simulink model "EV_Modeling_old"  (R2024b)
settings: Solver=FixedStepAuto  StartTime=0.0  StopTime=10382  FixedStep=0.1  RelTol=1e-3
values from neighbouring files (symbols this model uses):
  battery_SOC_SOC = battery_SOC(:,1)    [EV_Truck.m]    (also in simulink.m)
  battery_SOC_voltage = battery_SOC(:,2)    [EV_Truck.m]    (also in simulink.m)
  drag_coefficient_FV1 = table2array(drag_coefficient(:,3))    [simulink.m]
  drag_coefficient_FV2 = table2array(drag_coefficient(:,4))    [simulink.m]
  drag_coefficient_input = table2array(drag_coefficient(:,1))    [simulink.m]
  drag_coefficient_LV = table2array(drag_coefficient(:,2))    [simulink.m]
  electric_consumption_ressistancce = electric_consumption(:,2)    [EV_Truck.m]    (also in simulink.m)
  electric_consumption_voltage = electric_consumption(:,1)    [EV_Truck.m]    (also in simulink.m)
  motor_efficiency_efficiency = table2array(motor_efficiency(2:height(motor_efficiency),2:width(motor_efficiency)))    [EV_Truck.m]    (also in simulink.m)
  motor_efficiency_RPM = table2array(motor_efficiency(2:height(motor_efficiency),1))    [EV_Truck.m]    (also in simulink.m)
  motor_efficiency_torque = transpose(motor_efficiency_torque)    [EV_Truck.m]    (also in simulink.m)
  motor_RPM_torque = table2array(motor_torque(1:14,1))    [EV_Truck.m]    (also in simulink.m)
  motor_torque_RPM = table2array(motor_torque(1:14,2))    [EV_Truck.m]    (also in simulink.m)
undefined symbols (not defined in the file or in its folder): battery_builder_rtmsupport, battery_sli_rtmsupport, C1_mat, C2_mat, c_sqrt, DiscIntNeverNeededParam, dV0_mat, gcbh, n, Wc, Wm, x0
libraries: simulink x87, packLibrary_lib x30, nesl_utility x6, fl_lib x6, simulink_extras x3, mpcadaslib x2, slpidlib x1
(part 11 of 12)

== system EV_Modeling_old/FV2/SOC Estimator (Kalman Filter)1/Kalman Filter/UKF/Prediction/Measurement function ==
  Current : Inport
  Temperature : Inport  Port=2
  X : Inport  Port=3  Partition=on  PartitionDimension=2  PartitionWidth=1  PartitionOffset=0
  Constant : Constant  Value=Wm  OutDataTypeStr=Inherit: Inherit via back propagation
  Data Type Conversion Inherited : simulink/Signal Attributes/Data Type Conversion Inherited  ConvertRealWorld=Real World Value  DoSatur=off
  For Each : ForEach  DisableCoverage=on  ShowIterationIndex=on
  Measurement function : Subsystem
  Product : Product
  Selector : Selector  IndexMode=Zero-based  InputPortWidth=2*n+1  IndexOptions=Index vector (port)  Indices=[1 3]  OutputSizes=1
  y : Outport  ConcatenationDimension=2
  Wm_i*y_i : Outport  Port=2  SampleTime=Ts  ConcatenationDimension=2
  wires:
  Product/1 -> Wm_i*y_i/1
  Selector/1 -> Product/1
  For Each/1 -> Selector/2
  Measurement function/1(y) -> Product/2, y/1
  Temperature/1 -> Measurement function/2(Temperature)
  Current/1 -> Data Type Conversion Inherited/1, Measurement function/1(Current)
  X/1 -> Measurement function/3(x)
  Data Type Conversion Inherited/1 -> Selector/1
  Constant/1 -> Data Type Conversion Inherited/2

== system EV_Modeling_old/FV2/SOC Estimator (Kalman Filter)1/Kalman Filter/UKF/Prediction/State function ==
  Current : Inport
  Temperature : Inport  Port=2
  X : Inport  Port=3  Partition=on  PartitionDimension=2  PartitionWidth=1  PartitionOffset=0
  Constant : Constant  Value=Wm  OutDataTypeStr=Inherit: Inherit via back propagation
  Data Type Conversion Inherited : simulink/Signal Attributes/Data Type Conversion Inherited  ConvertRealWorld=Real World Value  DoSatur=off
  For Each : ForEach  DisableCoverage=on  ShowIterationIndex=on
  Product : Product
  Selector : Selector  IndexMode=Zero-based  InputPortWidth=2*n+1  IndexOptions=Index vector (port)  Indices=[1 3]  OutputSizes=1
  State function : Subsystem
  xk1 : Outport  ConcatenationDimension=2
  Wm_i*xk1_i : Outport  Port=2  SampleTime=Ts  ConcatenationDimension=2
  wires:
  X/1 -> State function/3(x)
  Current/1 -> Data Type Conversion Inherited/1, State function/1(Current)
  Temperature/1 -> State function/2(Temperature)
  State function/1(xk1) -> Product/2, xk1/1
  For Each/1 -> Selector/2
  Selector/1 -> Product/1
  Product/1 -> Wm_i*xk1_i/1
  Data Type Conversion Inherited/1 -> Selector/1
  Constant/1 -> Data Type Conversion Inherited/2

== system EV_Modeling_old/FV2/SOC Estimator (Kalman Filter)1/Kalman Filter/UKF 2RC/Prediction/Measurement function ==
  Current : Inport
  Temperature : Inport  Port=2
  X : Inport  Port=3  Partition=on  PartitionDimension=2  PartitionWidth=1  PartitionOffset=0
  Constant : Constant  Value=Wm  OutDataTypeStr=Inherit: Inherit via back propagation
  Data Type Conversion Inherited : simulink/Signal Attributes/Data Type Conversion Inherited  ConvertRealWorld=Real World Value  DoSatur=off
  For Each : ForEach  DisableCoverage=on  ShowIterationIndex=on
  Measurement function : Subsystem
  Product : Product
  Selector : Selector  IndexMode=Zero-based  InputPortWidth=2*n+1  IndexOptions=Index vector (port)  Indices=[1 3]  OutputSizes=1
  y : Outport  ConcatenationDimension=2
  Wm_i*y_i : Outport  Port=2  SampleTime=Ts  ConcatenationDimension=2
  wires:
  Product/1 -> Wm_i*y_i/1
  Selector/1 -> Product/1
  For Each/1 -> Selector/2
  Measurement function/1(y) -> Product/2, y/1
  Temperature/1 -> Measurement function/2(Temperature)
  Current/1 -> Data Type Conversion Inherited/1, Measurement function/1(Current)
  X/1 -> Measurement function/3(x)
  Data Type Conversion Inherited/1 -> Selector/1
  Constant/1 -> Data Type Conversion Inherited/2

== system EV_Modeling_old/FV2/SOC Estimator (Kalman Filter)1/Kalman Filter/UKF 2RC/Prediction/State function ==
  Current : Inport
  Temperature : Inport  Port=2
  X : Inport  Port=3  Partition=on  PartitionDimension=2  PartitionWidth=1  PartitionOffset=0
  Constant : Constant  Value=Wm  OutDataTypeStr=Inherit: Inherit via back propagation
  Data Type Conversion Inherited : simulink/Signal Attributes/Data Type Conversion Inherited  ConvertRealWorld=Real World Value  DoSatur=off
  For Each : ForEach  DisableCoverage=on  ShowIterationIndex=on
  Product : Product
  Selector : Selector  IndexMode=Zero-based  InputPortWidth=2*n+1  IndexOptions=Index vector (port)  Indices=[1 3]  OutputSizes=1
  State function : Subsystem
  xk1 : Outport  ConcatenationDimension=2
  Wm_i*xk1_i : Outport  Port=2  SampleTime=Ts  ConcatenationDimension=2
  wires:
  X/1 -> State function/3(x)
  Current/1 -> Data Type Conversion Inherited/1, State function/1(Current)
  Temperature/1 -> State function/2(Temperature)
  State function/1(xk1) -> Product/2, xk1/1
  For Each/1 -> Selector/2
  Selector/1 -> Product/1
  Product/1 -> Wm_i*xk1_i/1
  Data Type Conversion Inherited/1 -> Selector/1
  Constant/1 -> Data Type Conversion Inherited/2

== system EV_Modeling_old/LV/SOC Estimator (Kalman Filter)/Kalman Filter/UKBF/Prediction-correction/Measurement function ==
  Current : Inport
  Temperature : Inport  Port=2
  X : Inport  Port=3  Partition=on  PartitionDimension=2  PartitionWidth=1  PartitionOffset=0
  Constant : Constant  Value=Wm
  For Each : ForEach  DisableCoverage=on  ShowIterationIndex=on
  Measurement function : Subsystem
  Product : Product
  Selector : Selector  IndexMode=Zero-based  InputPortWidth=2*n+1  IndexOptions=Index vector (port)  Indices=[1 3]  OutputSizes=1
  h(X) : Outport  ConcatenationDimension=2
  h(X)*Wm : Outport  Port=2  ConcatenationDimension=2
  wires:
  Temperature/1 -> Measurement function/2(Temperature)
  Current/1 -> Measurement function/1(Current)
  X/1 -> Measurement function/3(x)
  For Each/1 -> Selector/2
  Constant/1 -> Selector/1
  Selector/1 -> Product/1
  Measurement function/1(y) -> Product/2, h(X)/1
  Product/1 -> h(X)*Wm/1

== system EV_Modeling_old/LV/SOC Estimator (Kalman Filter)/Kalman Filter/UKBF/Prediction-correction/State function ==
  Current : Inport
  Temperature : Inport  Port=2
  X : Inport  Port=3  Partition=on  PartitionDimension=2  PartitionWidth=1  PartitionOffset=0
  Constant : Constant  Value=double(Wm)
  For Each : ForEach  DisableCoverage=on  ShowIterationIndex=on
  Product : Product
  Product1 : Product
  Selector : Selector  IndexMode=Zero-based  InputPortWidth=2*n+1  IndexOptions=Index vector (port)  Indices=[1 3]  OutputSizes=1
  State function : Subsystem
  f(X) : Outport  ConcatenationDimension=2
  f(X)*Wm : Outport  Port=2  ConcatenationDimension=2
  X*Wm : Outport  Port=3  ConcatenationDimension=2
  wires:
  Current/1 -> State function/1(Current)
  Temperature/1 -> State function/2(Temperature)
  Constant/1 -> Selector/1
  Product/1 -> f(X)*Wm/1
  State function/1(f(x)) -> Product/2, f(X)/1
  Selector/1 -> Product1/1, Product/1
  For Each/1 -> Selector/2
  X/1 -> Product1/2, State function/3(x)
  Product1/1 -> X*Wm/1

== system EV_Modeling_old/LV/SOC Estimator (Kalman Filter)/Kalman Filter/UKBF/Prediction-correction/Update A ==
  X : Inport
  Constant : Constant  Value=ones(1,2*n+1)  VectorParams1D=off
  Gain : Gain  Gain=1/c_sqrt
  Matrix Multiply : Product  Multiplication=Matrix(*)
  Selector : Selector  NumberOfDimensions=2  InputPortWidth=3  IndexOptions=Index vector (dialog),Index vector (dialog)  Indices=[1:n],1  OutputSizes=1,1
  Selector1 : Selector  NumberOfDimensions=2  InputPortWidth=3  IndexOptions=Index vector (dialog),Index vector (dialog)  Indices=1:n,2:n+1  OutputSizes=1,1
  Sum : Sum  Inputs=|+-
  A(t) : Outport
  xhat : Outport  Port=2
  wires:
  X/1 -> Selector/1, Sum/1
  Selector/1 -> xhat/1, Matrix Multiply/1
  Constant/1 -> Matrix Multiply/2
  Matrix Multiply/1 -> Sum/2
  Sum/1 -> Gain/1
  Gain/1 -> Selector1/1
  Selector1/1 -> A(t)/1

== system EV_Modeling_old/LV/SOC Estimator (Kalman Filter)/Kalman Filter/UKBF/Prediction-correction/Xdot ==
  Voltage : Inport
  h(X) : Inport  Port=2
  mh : Inport  Port=3
  f(X) : Inport  Port=4
  mf : Inport  Port=5
  mx : Inport  Port=6
  X : Inport  Port=7
  A : Inport  Port=8
  Constant : Constant  Value=ones(1,2*n+1)  VectorParams1D=off
  Constant2 : Constant  Value=double(R)
  Constant3 : Constant  Value=eye(size(R,1))
  Divide : Product  Inputs=*/  Multiplication=Matrix(*)
  Gain3 : Gain  Gain=[Wc;Wc]
  Gain4 : Gain  Gain=[Wc;Wc]
  Matrix Multiply{,1..6,9} (8 alike) : Product  Multiplication=Matrix(*)
  Sigma points derivatives : Subsystem
  Sum : Sum  Inputs=|+-
  Sum1 : Sum  Inputs=|+-
  Sum2 : Sum  Inputs=|+-
  Sum4 : Sum  Inputs=-+|
  Sum5 : Sum
  Transpose : Math  Operator=transpose
  Transpose1 : Math  Operator=transpose
  Transpose2 : Math  Operator=transpose
  Update Fi : Subsystem
  Xdot : Outport
  wires:
  Constant/1 -> Matrix Multiply/2, Matrix Multiply1/2, Matrix Multiply2/2
  X/1 -> Sum/1
  f(X)/1 -> Sum1/1
  mf/1 -> Matrix Multiply1/1, Sum5/1
  h(X)/1 -> Sum2/1
  mh/1 -> Sum4/1, Matrix Multiply2/1
  Matrix Multiply/1 -> Sum/2
  Matrix Multiply1/1 -> Sum1/2
  Sum1/1 -> Gain4/1, Transpose/1
  Transpose/1 -> Matrix Multiply3/2
  Gain3/1 -> Matrix Multiply5/1, Matrix Multiply3/1
  Matrix Multiply2/1 -> Sum2/2
  Gain4/1 -> Matrix Multiply4/1
  Sum/1 -> Transpose1/1, Gain3/1
  Transpose1/1 -> Matrix Multiply4/2
  Sum2/1 -> Transpose2/1
  Transpose2/1 -> Matrix Multiply5/2
  Matrix Multiply5/1 -> Matrix Multiply6/1  "XWh"
  Constant2/1 -> Divide/2
  Constant3/1 -> Divide/1
  Divide/1 -> Matrix Multiply6/2
  Matrix Multiply6/1 -> Update Fi/4(K), Matrix Multiply9/1  "K"
  Voltage/1 -> Sum4/2
  Sum4/1 -> Matrix Multiply9/2
  Matrix Multiply9/1 -> Sum5/2
  Sum5/1 -> Sigma points derivatives/3(x1)
  A/1 -> Sigma points derivatives/1(A), Update Fi/1(A)
  Matrix Multiply3/1 -> Update Fi/2(XWf)  "XWf"
  Matrix Multiply4/1 -> Update Fi/3(fWX)  "fWX"
  Sigma points derivatives/1(Xdot) -> Xdot/1
  Update Fi/1(Fi) -> Sigma points derivatives/2(Fi)
  mx/1 -> Matrix Multiply/1

== system EV_Modeling_old/LV/SOC Estimator (Kalman Filter)/Kalman Filter/UKBF 2RC/Prediction-correction/Measurement function ==
  Current : Inport
  Temperature : Inport  Port=2
  X : Inport  Port=3  Partition=on  PartitionDimension=2  PartitionWidth=1  PartitionOffset=0
  Constant : Constant  Value=Wm
  For Each : ForEach  DisableCoverage=on  ShowIterationIndex=on
  Measurement function : Subsystem
  Product : Product
  Selector : Selector  IndexMode=Zero-based  InputPortWidth=2*n+1  IndexOptions=Index vector (port)  Indices=[1 3]  OutputSizes=1
  h(X) : Outport  ConcatenationDimension=2
  h(X)*Wm : Outport  Port=2  ConcatenationDimension=2
  wires:
  Temperature/1 -> Measurement function/2(Temperature)
  Current/1 -> Measurement function/1(Current)
  X/1 -> Measurement function/3(x)
  For Each/1 -> Selector/2
  Constant/1 -> Selector/1
  Selector/1 -> Product/1
  Measurement function/1(y) -> Product/2, h(X)/1
  Product/1 -> h(X)*Wm/1

== system EV_Modeling_old/LV/SOC Estimator (Kalman Filter)/Kalman Filter/UKBF 2RC/Prediction-correction/State function ==
  Current : Inport
  Temperature : Inport  Port=2
  X : Inport  Port=3  Partition=on  PartitionDimension=2  PartitionWidth=1  PartitionOffset=0
  Constant : Constant  Value=double(Wm)
  For Each : ForEach  DisableCoverage=on  ShowIterationIndex=on
  Product : Product
  Product1 : Product
  Selector : Selector  IndexMode=Zero-based  InputPortWidth=2*n+1  IndexOptions=Index vector (port)  Indices=[1 3]  OutputSizes=1
  State function : Subsystem
  f(X) : Outport  ConcatenationDimension=2
  f(X)*Wm : Outport  Port=2  ConcatenationDimension=2
  X*Wm : Outport  Port=3  ConcatenationDimension=2
  wires:
  Current/1 -> State function/1(Current)
  Temperature/1 -> State function/2(Temperature)
  Constant/1 -> Selector/1
  Product/1 -> f(X)*Wm/1
  State function/1(f(x)) -> Product/2, f(X)/1
  Selector/1 -> Product1/1, Product/1
  For Each/1 -> Selector/2
  X/1 -> Product1/2, State function/3(x)
  Product1/1 -> X*Wm/1

== system EV_Modeling_old/LV/SOC Estimator (Kalman Filter)/Kalman Filter/UKBF 2RC/Prediction-correction/Update A ==
  X : Inport
  Constant : Constant  Value=ones(1,2*n+1)  VectorParams1D=off
  Gain : Gain  Gain=1/c_sqrt
  Matrix Multiply : Product  Multiplication=Matrix(*)
  Selector : Selector  NumberOfDimensions=2  InputPortWidth=3  IndexOptions=Index vector (dialog),Index vector (dialog)  Indices=[1:n],1  OutputSizes=1,1
  Selector1 : Selector  NumberOfDimensions=2  InputPortWidth=3  IndexOptions=Index vector (dialog),Index vector (dialog)  Indices=1:n,2:n+1  OutputSizes=1,1
  Sum : Sum  Inputs=|+-
  A(t) : Outport
  xhat : Outport  Port=2
  wires:
  X/1 -> Selector/1, Sum/1
  Selector/1 -> xhat/1, Matrix Multiply/1
  Constant/1 -> Matrix Multiply/2
  Matrix Multiply/1 -> Sum/2
  Sum/1 -> Gain/1
  Gain/1 -> Selector1/1
  Selector1/1 -> A(t)/1

== system EV_Modeling_old/LV/SOC Estimator (Kalman Filter)/Kalman Filter/UKBF 2RC/Prediction-correction/Xdot ==
  Voltage : Inport
  h(X) : Inport  Port=2
  mh : Inport  Port=3
  f(X) : Inport  Port=4
  mf : Inport  Port=5
  mx : Inport  Port=6
  X : Inport  Port=7
  A : Inport  Port=8
  Constant : Constant  Value=ones(1,2*n+1)  VectorParams1D=off
  Constant2 : Constant  Value=double(R)
  Constant3 : Constant  Value=eye(size(R,1))
  Divide : Product  Inputs=*/  Multiplication=Matrix(*)
  Gain3 : Gain  Gain=[Wc;Wc;Wc]
  Gain4 : Gain  Gain=[Wc;Wc;Wc]
  Matrix Multiply{,1..6,9} (8 alike) : Product  Multiplication=Matrix(*)
  Sigma points derivatives : Subsystem
  Sum : Sum  Inputs=|+-
  Sum1 : Sum  Inputs=|+-
  Sum2 : Sum  Inputs=|+-
  Sum4 : Sum  Inputs=-+|
  Sum5 : Sum
  Transpose : Math  Operator=transpose
  Transpose1 : Math  Operator=transpose
  Transpose2 : Math  Operator=transpose
  Update Fi : Subsystem
  Xdot : Outport
  wires:
  Constant/1 -> Matrix Multiply/2, Matrix Multiply1/2, Matrix Multiply2/2
  X/1 -> Sum/1
  f(X)/1 -> Sum1/1
  mf/1 -> Matrix Multiply1/1, Sum5/1
  h(X)/1 -> Sum2/1
  mh/1 -> Sum4/1, Matrix Multiply2/1
  Matrix Multiply/1 -> Sum/2
  Matrix Multiply1/1 -> Sum1/2
  Sum1/1 -> Gain4/1, Transpose/1
  Transpose/1 -> Matrix Multiply3/2
  Gain3/1 -> Matrix Multiply5/1, Matrix Multiply3/1
  Matrix Multiply2/1 -> Sum2/2
  Gain4/1 -> Matrix Multiply4/1
  Sum/1 -> Transpose1/1, Gain3/1
  Transpose1/1 -> Matrix Multiply4/2
  Sum2/1 -> Transpose2/1
  Transpose2/1 -> Matrix Multiply5/2
  Matrix Multiply5/1 -> Matrix Multiply6/1  "XWh"
  Constant2/1 -> Divide/2
  Constant3/1 -> Divide/1
  Divide/1 -> Matrix Multiply6/2
  Matrix Multiply6/1 -> Update Fi/4(K), Matrix Multiply9/1  "K"
  Voltage/1 -> Sum4/2
  Sum4/1 -> Matrix Multiply9/2
  Matrix Multiply9/1 -> Sum5/2
  Sum5/1 -> Sigma points derivatives/3(x1)
  A/1 -> Sigma points derivatives/1(A), Update Fi/1(A)
  Matrix Multiply3/1 -> Update Fi/2(XWf)  "XWf"
  Matrix Multiply4/1 -> Update Fi/3(fWX)  "fWX"
  Sigma points derivatives/1(Xdot) -> Xdot/1
  Update Fi/1(Fi) -> Sigma points derivatives/2(Fi)
  mx/1 -> Matrix Multiply/1

== system EV_Modeling_old/LV/SOC Estimator (Kalman Filter)/Kalman Filter/UKF/Prediction/Measurement function ==
  Current : Inport
  Temperature : Inport  Port=2
  X : Inport  Port=3  Partition=on  PartitionDimension=2  PartitionWidth=1  PartitionOffset=0
  Constant : Constant  Value=Wm  OutDataTypeStr=Inherit: Inherit via back propagation
  Data Type Conversion Inherited : simulink/Signal Attributes/Data Type Conversion Inherited  ConvertRealWorld=Real World Value  DoSatur=off
  For Each : ForEach  DisableCoverage=on  ShowIterationIndex=on
  Measurement function : Subsystem
  Product : Product
  Selector : Selector  IndexMode=Zero-based  InputPortWidth=2*n+1  IndexOptions=Index vector (port)  Indices=[1 3]  OutputSizes=1
  y : Outport  ConcatenationDimension=2
  Wm_i*y_i : Outport  Port=2  SampleTime=Ts  ConcatenationDimension=2
  wires:
  Product/1 -> Wm_i*y_i/1
  Selector/1 -> Product/1
  For Each/1 -> Selector/2
  Measurement function/1(y) -> Product/2, y/1
  Temperature/1 -> Measurement function/2(Temperature)
  Current/1 -> Data Type Conversion Inherited/1, Measurement function/1(Current)
  X/1 -> Measurement function/3(x)
  Data Type Conversion Inherited/1 -> Selector/1
  Constant/1 -> Data Type Conversion Inherited/2

== system EV_Modeling_old/LV/SOC Estimator (Kalman Filter)/Kalman Filter/UKF/Prediction/State function ==
  Current : Inport
  Temperature : Inport  Port=2
  X : Inport  Port=3  Partition=on  PartitionDimension=2  PartitionWidth=1  PartitionOffset=0
  Constant : Constant  Value=Wm  OutDataTypeStr=Inherit: Inherit via back propagation
  Data Type Conversion Inherited : simulink/Signal Attributes/Data Type Conversion Inherited  ConvertRealWorld=Real World Value  DoSatur=off
  For Each : ForEach  DisableCoverage=on  ShowIterationIndex=on
  Product : Product
  Selector : Selector  IndexMode=Zero-based  InputPortWidth=2*n+1  IndexOptions=Index vector (port)  Indices=[1 3]  OutputSizes=1
  State function : Subsystem
  xk1 : Outport  ConcatenationDimension=2
  Wm_i*xk1_i : Outport  Port=2  SampleTime=Ts  ConcatenationDimension=2
  wires:
  X/1 -> State function/3(x)
  Current/1 -> Data Type Conversion Inherited/1, State function/1(Current)
  Temperature/1 -> State function/2(Temperature)
  State function/1(xk1) -> Product/2, xk1/1
  For Each/1 -> Selector/2
  Selector/1 -> Product/1
  Product/1 -> Wm_i*xk1_i/1
  Data Type Conversion Inherited/1 -> Selector/1
  Constant/1 -> Data Type Conversion Inherited/2

== system EV_Modeling_old/LV/SOC Estimator (Kalman Filter)/Kalman Filter/UKF 2RC/Prediction/Measurement function ==
  Current : Inport
  Temperature : Inport  Port=2
  X : Inport  Port=3  Partition=on  PartitionDimension=2  PartitionWidth=1  PartitionOffset=0
  Constant : Constant  Value=Wm  OutDataTypeStr=Inherit: Inherit via back propagation
  Data Type Conversion Inherited : simulink/Signal Attributes/Data Type Conversion Inherited  ConvertRealWorld=Real World Value  DoSatur=off
  For Each : ForEach  DisableCoverage=on  ShowIterationIndex=on
  Measurement function : Subsystem
  Product : Product
  Selector : Selector  IndexMode=Zero-based  InputPortWidth=2*n+1  IndexOptions=Index vector (port)  Indices=[1 3]  OutputSizes=1
  y : Outport  ConcatenationDimension=2
  Wm_i*y_i : Outport  Port=2  SampleTime=Ts  ConcatenationDimension=2
  wires:
  Product/1 -> Wm_i*y_i/1
  Selector/1 -> Product/1
  For Each/1 -> Selector/2
  Measurement function/1(y) -> Product/2, y/1
  Temperature/1 -> Measurement function/2(Temperature)
  Current/1 -> Data Type Conversion Inherited/1, Measurement function/1(Current)
  X/1 -> Measurement function/3(x)
  Data Type Conversion Inherited/1 -> Selector/1
  Constant/1 -> Data Type Conversion Inherited/2

== system EV_Modeling_old/LV/SOC Estimator (Kalman Filter)/Kalman Filter/UKF 2RC/Prediction/State function ==
  Current : Inport
  Temperature : Inport  Port=2
  X : Inport  Port=3  Partition=on  PartitionDimension=2  PartitionWidth=1  PartitionOffset=0
  Constant : Constant  Value=Wm  OutDataTypeStr=Inherit: Inherit via back propagation
  Data Type Conversion Inherited : simulink/Signal Attributes/Data Type Conversion Inherited  ConvertRealWorld=Real World Value  DoSatur=off
  For Each : ForEach  DisableCoverage=on  ShowIterationIndex=on
  Product : Product
  Selector : Selector  IndexMode=Zero-based  InputPortWidth=2*n+1  IndexOptions=Index vector (port)  Indices=[1 3]  OutputSizes=1
  State function : Subsystem
  xk1 : Outport  ConcatenationDimension=2
  Wm_i*xk1_i : Outport  Port=2  SampleTime=Ts  ConcatenationDimension=2
  wires:
  X/1 -> State function/3(x)
  Current/1 -> Data Type Conversion Inherited/1, State function/1(Current)
  Temperature/1 -> State function/2(Temperature)
  State function/1(xk1) -> Product/2, xk1/1
  For Each/1 -> Selector/2
  Selector/1 -> Product/1
  Product/1 -> Wm_i*xk1_i/1
  Data Type Conversion Inherited/1 -> Selector/1
  Constant/1 -> Data Type Conversion Inherited/2

== system EV_Modeling_old/FV1/SOC Estimator (Kalman Filter)1/Kalman Filter/UKBF/Prediction-correction/Measurement function/Measurement function ==
  Current : Inport
  Temperature : Inport  Port=2
  x : Inport  Port=3
  Add2 : Sum  Inputs=+--
  Get SOC1 : Selector  InputPortWidth=2  IndexOptions=Index vector (dialog)  Indices=[1]  OutputSizes=1
  Get V1 : Selector  InputPortWidth=2  IndexOptions=Index vector (dialog)  Indices=2  OutputSizes=1
  OCV Table : Lookup_n-D  BreakpointsForDimension1=SOC_vec  BreakpointsForDimension2=T_vec  BeginIndexSearchUsingPreviousIndexResult=on  Table=V0_mat  ExtrapMethod=Clip  InternalRulePriority=Speed  RndMeth=Simplest
      settings: InputPortMap=u0,u1
  Product2 : Product
  R0 Table : Lookup_n-D  BreakpointsForDimension1=SOC_vec  BreakpointsForDimension2=T_vec  BeginIndexSearchUsingPreviousIndexResult=on  Table=R0_mat  ExtrapMethod=Clip  InternalRulePriority=Speed  RndMeth=Simplest
      settings: InputPortMap=u0,u1
  y : Outport
  wires:
  x/1 -> Get SOC1/1, Get V1/1
  OCV Table/1 -> Add2/1
  Current/1 -> Product2/2
  Get SOC1/1 -> OCV Table/1, R0 Table/1  "SOC"
  Get V1/1 -> Add2/3
  Product2/1 -> Add2/2
  Add2/1 -> y/1
  R0 Table/1 -> Product2/1
  Temperature/1 -> R0 Table/2, OCV Table/2

== system EV_Modeling_old/FV1/SOC Estimator (Kalman Filter)1/Kalman Filter/UKBF/Prediction-correction/State function/State function ==
  Current : Inport
  Temperature : Inport  Port=2
  x : Inport  Port=3
  Add1 : Sum  Inputs=-+
  C1 : Lookup_n-D  BreakpointsForDimension1=SOC_vec  BreakpointsForDimension2=T_vec  BeginIndexSearchUsingPreviousIndexResult=on  Table=C1_mat  ExtrapMethod=Clip  InternalRulePriority=Speed  RndMeth=Simplest
      settings: InputPortMap=u0,u1
  Divide1 : Product  Inputs=*/
  Divide2 : Product  Inputs=*/
  Gain : Gain  Gain=-1/(AH*3600)
  Get SOC : Selector  InputPortWidth=2  IndexOptions=Index vector (dialog)  Indices=1  OutputSizes=1
  Get V1 : Selector  InputPortWidth=2  IndexOptions=Index vector (dialog)  Indices=2  OutputSizes=1
  Mux : Mux  Inputs=2
  Product1 : Product
  R1 : Lookup_n-D  BreakpointsForDimension1=SOC_vec  BreakpointsForDimension2=T_vec  BeginIndexSearchUsingPreviousIndexResult=on  Table=R1_mat  ExtrapMethod=Clip  InternalRulePriority=Speed  RndMeth=Simplest
      settings: InputPortMap=u0,u1
  f(x) : Outport
  wires:
  Gain/1 -> Mux/1
  Temperature/1 -> R1/2, C1/2
  x/1 -> Get SOC/1, Get V1/1
  Add1/1 -> Mux/2  "xdot_2"
  Divide2/1 -> Add1/1
  Mux/1 -> f(x)/1  "xdot"
  Current/1 -> Divide1/1, Gain/1  "Current"
  C1/1 -> Divide1/2, Product1/2  "C1"
  Get V1/1 -> Divide2/1  "V1"
  R1/1 -> Product1/1  "R1"
  Get SOC/1 -> R1/1, C1/1
  Product1/1 -> Divide2/2  "R1*C1"
  Divide1/1 -> Add1/2  "Current/C1"

== system EV_Modeling_old/FV1/SOC Estimator (Kalman Filter)1/Kalman Filter/UKBF/Prediction-correction/Xdot/Sigma points derivatives ==
  A : Inport
  Fi : Inport  Port=2
  x1 : Inport  Port=3
  Assignment : Assignment  NumberOfDimensions=2  DiagnosticForDimensions=Warning  IndexOptions=Index vector (dialog),Index vector (dialog)  Indices=1:n,1  OutputSizes=1,1
  Assignment1 : Assignment  NumberOfDimensions=2  DiagnosticForDimensions=Warning  IndexOptions=Index vector (dialog),Index vector (dialog)  Indices=1:n,2:n+1  OutputSizes=1,1
  Assignment2 : Assignment  NumberOfDimensions=2  DiagnosticForDimensions=Warning  IndexOptions=Index vector (dialog),Index vector (dialog)  Indices=1:n,n+2:2*n+1  OutputSizes=1,1
  Constant : Constant  Value=zeros(n,2*n+1)
  Constant1 : Constant  Value=ones(1,n)  VectorParams1D=off
  Gain : Gain  Gain=c_sqrt
  Matrix Multiply : Product  Multiplication=Matrix(*)
  Matrix Multiply1 : Product  Multiplication=Matrix(*)
  Sum : Sum  Inputs=|++
  Sum1 : Sum  Inputs=|+-
  Xdot : Outport
  wires:
  x1/1 -> Matrix Multiply/1, Assignment/2
  Constant1/1 -> Matrix Multiply/2
  Matrix Multiply/1 -> Sum1/1, Sum/1
  Gain/1 -> Sum1/2, Sum/2
  Sum/1 -> Assignment1/2
  Sum1/1 -> Assignment2/2
  Constant/1 -> Assignment/1
  Assignment/1 -> Assignment1/1
  Assignment1/1 -> Assignment2/1
  Assignment2/1 -> Xdot/1
  A/1 -> Matrix Multiply1/1
  Fi/1 -> Matrix Multiply1/2
  Matrix Multiply1/1 -> Gain/1

== system EV_Modeling_old/FV1/SOC Estimator (Kalman Filter)1/Kalman Filter/UKBF/Prediction-correction/Xdot/Update Fi ==
  A : Inport
  XWf : Inport  Port=2
  fWX : Inport  Port=3
  K : Inport  Port=4
  Constant1 : Constant  Value=double(Q)
  Constant4 : Constant  Value=eye(size(P0,1))
  Constant5 : Constant  Value=double(R)
  Divide1 : Product  Inputs=*/  Multiplication=Matrix(*)
  Gain5 : Gain  Gain=tril(ones(n)-diag(0.5*ones(1,n)))
  Matrix Multiply7 : Product  Inputs=3  Multiplication=Matrix(*)
  Matrix Multiply8 : Product  Inputs=3  Multiplication=Matrix(*)
  Sum3 : Sum  Inputs=+++-
  Transpose3 : Math  Operator=transpose
  Transpose4 : Math  Operator=transpose
  Fi : Outport
  wires:
  A/1 -> Divide1/2
  Matrix Multiply7/1 -> Gain5/1  "M"
  Constant1/1 -> Sum3/3
  Sum3/1 -> Matrix Multiply7/2
  Transpose3/1 -> Matrix Multiply8/3
  Matrix Multiply8/1 -> Sum3/4
  Divide1/1 -> Transpose4/1, Matrix Multiply7/1
  K/1 -> Transpose3/1, Matrix Multiply8/1
  XWf/1 -> Sum3/1
  Constant4/1 -> Divide1/1
  Transpose4/1 -> Matrix Multiply7/3
  Constant5/1 -> Matrix Multiply8/2
  fWX/1 -> Sum3/2
  Gain5/1 -> Fi/1  "Fi"

== system EV_Modeling_old/FV1/SOC Estimator (Kalman Filter)1/Kalman Filter/UKBF 2RC/Prediction-correction/Measurement function/Measurement function ==
  Current : Inport
  Temperature : Inport  Port=2
  x : Inport  Port=3
  Add2 : Sum  Inputs=+---
  Get SOC1 : Selector  InputPortWidth=3  IndexOptions=Index vector (dialog)  Indices=[1]  OutputSizes=1
  Get V1 : Selector  InputPortWidth=3  IndexOptions=Index vector (dialog)  Indices=2  OutputSizes=1
  Get V2 : Selector  InputPortWidth=3  IndexOptions=Index vector (dialog)  Indices=3  OutputSizes=1
  OCV Table : Lookup_n-D  BreakpointsForDimension1=SOC_vec  BreakpointsForDimension2=T_vec  BeginIndexSearchUsingPreviousIndexResult=on  Table=V0_mat  ExtrapMethod=Clip  InternalRulePriority=Speed  RndMeth=Simplest
      settings: InputPortMap=u0,u1
  Product2 : Product
  R0 Table : Lookup_n-D  BreakpointsForDimension1=SOC_vec  BreakpointsForDimension2=T_vec  BeginIndexSearchUsingPreviousIndexResult=on  Table=R0_mat  ExtrapMethod=Clip  InternalRulePriority=Speed  RndMeth=Simplest
      settings: InputPortMap=u0,u1
  y : Outport
  wires:
  Get V2/1 -> Add2/4
  x/1 -> Get SOC1/1, Get V1/1, Get V2/1
  OCV Table/1 -> Add2/1
  Current/1 -> Product2/2
  Get SOC1/1 -> OCV Table/1, R0 Table/1  "SOC"
  Get V1/1 -> Add2/3
  Product2/1 -> Add2/2
  Add2/1 -> y/1
  R0 Table/1 -> Product2/1
  Temperature/1 -> R0 Table/2, OCV Table/2

== system EV_Modeling_old/FV1/SOC Estimator (Kalman Filter)1/Kalman Filter/UKBF 2RC/Prediction-correction/State function/State function ==
  Current : Inport
  Temperature : Inport  Port=2
  x : Inport  Port=3
  2-D Lookup Table C2 : Lookup_n-D  BreakpointsForDimension1=SOC_vec  BreakpointsForDimension2=T_vec  Table=C2_mat  InternalRulePriority=Speed  RndMeth=Simplest
      settings: InputPortMap=u0,u1
  2-D Lookup Table R2 : Lookup_n-D  BreakpointsForDimension1=SOC_vec  BreakpointsForDimension2=T_vec  Table=R2_mat  InternalRulePriority=Speed  RndMeth=Simplest
      settings: InputPortMap=u0,u1
  Add1 : Sum  Inputs=-+
  Add2 : Sum  Inputs=-+
  C1 : Lookup_n-D  BreakpointsForDimension1=SOC_vec  BreakpointsForDimension2=T_vec  BeginIndexSearchUsingPreviousIndexResult=on  Table=C1_mat  ExtrapMethod=Clip  InternalRulePriority=Speed  RndMeth=Simplest
      settings: InputPortMap=u0,u1
  Divide{1..4} (4 alike) : Product  Inputs=*/
  Gain : Gain  Gain=-1/(AH*3600)
  Get SOC : Selector  InputPortWidth=3  IndexOptions=Index vector (dialog)  Indices=1  OutputSizes=1
  Get V1 : Selector  InputPortWidth=3  IndexOptions=Index vector (dialog)  Indices=2  OutputSizes=1
  Get V2 : Selector  InputPortWidth=3  IndexOptions=Index vector (dialog)  Indices=3  OutputSizes=1
  Mux : Mux  Inputs=3
  Product1 : Product
  Product2 : Product
  R1 : Lookup_n-D  BreakpointsForDimension1=SOC_vec  BreakpointsForDimension2=T_vec  BeginIndexSearchUsingPreviousIndexResult=on  Table=R1_mat  ExtrapMethod=Clip  InternalRulePriority=Speed  RndMeth=Simplest
      settings: InputPortMap=u0,u1
  f(x) : Outport
  wires:
  Divide4/1 -> Add2/2  "Current/C2"
  Divide3/1 -> Add2/1
  Add2/1 -> Mux/3  "xdot_3"
  Product2/1 -> Divide3/2  "R1*C1"
  Get V2/1 -> Divide3/1  "V2"
  2-D Lookup Table C2/1 -> Product2/2, Divide4/2  "C2"
  2-D Lookup Table R2/1 -> Product2/1  "R2"
  Gain/1 -> Mux/1
  Temperature/1 -> R1/2, C1/2, 2-D Lookup Table R2/2, 2-D Lookup Table C2/2
  x/1 -> Get SOC/1, Get V1/1, Get V2/1
  Add1/1 -> Mux/2  "xdot_2"
  Divide2/1 -> Add1/1
  Mux/1 -> f(x)/1  "xdot"
  Current/1 -> Divide1/1, Gain/1, Divide4/1  "Current"
  C1/1 -> Divide1/2, Product1/2  "C1"
  Get V1/1 -> Divide2/1  "V1"
  R1/1 -> Product1/1  "R1"
  Get SOC/1 -> R1/1, C1/1, 2-D Lookup Table R2/1, 2-D Lookup Table C2/1
  Product1/1 -> Divide2/2  "R1*C1"
  Divide1/1 -> Add1/2  "Current/C1"

== system EV_Modeling_old/FV1/SOC Estimator (Kalman Filter)1/Kalman Filter/UKBF 2RC/Prediction-correction/Xdot/Sigma points derivatives ==
  A : Inport
  Fi : Inport  Port=2
  x1 : Inport  Port=3
  Assignment : Assignment  NumberOfDimensions=2  DiagnosticForDimensions=Warning  IndexOptions=Index vector (dialog),Index vector (dialog)  Indices=1:n,1  OutputSizes=1,1
  Assignment1 : Assignment  NumberOfDimensions=2  DiagnosticForDimensions=Warning  IndexOptions=Index vector (dialog),Index vector (dialog)  Indices=1:n,2:n+1  OutputSizes=1,1
  Assignment2 : Assignment  NumberOfDimensions=2  DiagnosticForDimensions=Warning  IndexOptions=Index vector (dialog),Index vector (dialog)  Indices=1:n,n+2:2*n+1  OutputSizes=1,1
  Constant : Constant  Value=zeros(n,2*n+1)
  Constant1 : Constant  Value=ones(1,n)  VectorParams1D=off
  Gain : Gain  Gain=c_sqrt
  Matrix Multiply : Product  Multiplication=Matrix(*)
  Matrix Multiply1 : Product  Multiplication=Matrix(*)
  Sum : Sum  Inputs=|++
  Sum1 : Sum  Inputs=|+-
  Xdot : Outport
  wires:
  x1/1 -> Matrix Multiply/1, Assignment/2
  Constant1/1 -> Matrix Multiply/2
  Matrix Multiply/1 -> Sum1/1, Sum/1
  Gain/1 -> Sum1/2, Sum/2
  Sum/1 -> Assignment1/2
  Sum1/1 -> Assignment2/2
  Constant/1 -> Assignment/1
  Assignment/1 -> Assignment1/1
  Assignment1/1 -> Assignment2/1
  Assignment2/1 -> Xdot/1
  A/1 -> Matrix Multiply1/1
  Fi/1 -> Matrix Multiply1/2
  Matrix Multiply1/1 -> Gain/1

== system EV_Modeling_old/FV1/SOC Estimator (Kalman Filter)1/Kalman Filter/UKBF 2RC/Prediction-correction/Xdot/Update Fi ==
  A : Inport
  XWf : Inport  Port=2
  fWX : Inport  Port=3
  K : Inport  Port=4
  Constant1 : Constant  Value=double(Q_2RC)
  Constant4 : Constant  Value=eye(size(P0_2RC,1))
  Constant5 : Constant  Value=double(R)
  Divide1 : Product  Inputs=*/  Multiplication=Matrix(*)
  Gain5 : Gain  Gain=tril(ones(n)-diag(0.5*ones(1,n)))
  Matrix Multiply7 : Product  Inputs=3  Multiplication=Matrix(*)
  Matrix Multiply8 : Product  Inputs=3  Multiplication=Matrix(*)
  Sum3 : Sum  Inputs=+++-
  Transpose3 : Math  Operator=transpose
  Transpose4 : Math  Operator=transpose
  Fi : Outport
  wires:
  A/1 -> Divide1/2
  Matrix Multiply7/1 -> Gain5/1  "M"
  Constant1/1 -> Sum3/3
  Sum3/1 -> Matrix Multiply7/2
  Transpose3/1 -> Matrix Multiply8/3
  Matrix Multiply8/1 -> Sum3/4
  Divide1/1 -> Transpose4/1, Matrix Multiply7/1
  K/1 -> Transpose3/1, Matrix Multiply8/1
  XWf/1 -> Sum3/1
  Constant4/1 -> Divide1/1
  Transpose4/1 -> Matrix Multiply7/3
  Constant5/1 -> Matrix Multiply8/2
  fWX/1 -> Sum3/2
  Gain5/1 -> Fi/1  "Fi"

== system EV_Modeling_old/FV1/SOC Estimator (Kalman Filter)1/Kalman Filter/UKF/Prediction/Measurement function/Measurement function ==
  Current : Inport
  Temperature : Inport  Port=2
  x : Inport  Port=3
  Add2 : Sum  Inputs=+--
  Get SOC : Selector  InputPortWidth=2  IndexOptions=Index vector (dialog)  Indices=[1]  OutputSizes=1
  Get V1 : Selector  InputPortWidth=2  IndexOptions=Index vector (dialog)  Indices=2  OutputSizes=1
  OCV Table : Lookup_n-D  BreakpointsForDimension1=SOC_vec  BreakpointsForDimension2=T_vec  BeginIndexSearchUsingPreviousIndexResult=on  Table=V0_mat  ExtrapMethod=Clip  InternalRulePriority=Speed  RndMeth=Simplest
      settings: InputPortMap=u0,u1
  Product2 : Product
  R0 Table : Lookup_n-D  BreakpointsForDimension1=SOC_vec  BreakpointsForDimension2=T_vec  BeginIndexSearchUsingPreviousIndexResult=on  Table=R0_mat  ExtrapMethod=Clip  InternalRulePriority=Speed  RndMeth=Simplest
      settings: InputPortMap=u0,u1
  y : Outport
  wires:
  x/1 -> Get SOC/1, Get V1/1
  OCV Table/1 -> Add2/1
  Current/1 -> Product2/2
  Get SOC/1 -> OCV Table/1, R0 Table/1
  Get V1/1 -> Add2/3  "U1"
  Product2/1 -> Add2/2
  Add2/1 -> y/1
  R0 Table/1 -> Product2/1
  Temperature/1 -> R0 Table/2, OCV Table/2

== system EV_Modeling_old/FV1/SOC Estimator (Kalman Filter)1/Kalman Filter/UKF/Prediction/State function/State function ==
  Current : Inport
  Temperature : Inport  Port=2
  x : Inport  Port=3
  Add : Sum
  Add1 : Sum  Inputs=-+
  C1 : Lookup_n-D  BreakpointsForDimension1=SOC_vec  BreakpointsForDimension2=T_vec  BeginIndexSearchUsingPreviousIndexResult=on  Table=C1_mat  ExtrapMethod=Clip  InternalRulePriority=Speed  RndMeth=Simplest
      settings: InputPortMap=u0,u1
  Divide1 : Product  Inputs=*/
  Divide2 : Product  Inputs=*/
  Gain : Gain  Gain=-1/(AH*3600)
  Get SOC : Selector  InputPortWidth=2  IndexOptions=Index vector (dialog)  Indices=1  OutputSizes=1
  Get V1 : Selector  InputPortWidth=2  IndexOptions=Index vector (dialog)  Indices=2  OutputSizes=1
  Mux : Mux  Inputs=2
  Probe : Probe  ProbeWidth=off  ProbeComplexSignal=off  ProbeSampleTimeDataType=Same as input
  Product : Product  OutDataTypeStr=single
  Product1 : Product
  R1 : Lookup_n-D  BreakpointsForDimension1=SOC_vec  BreakpointsForDimension2=T_vec  BeginIndexSearchUsingPreviousIndexResult=on  Table=R1_mat  ExtrapMethod=Clip  InternalRulePriority=Speed  RndMeth=Simplest
      settings: InputPortMap=u0,u1
  Selector : Selector  InputPortWidth=2  IndexOptions=Index vector (dialog)  Indices=1  OutputSizes=1
  xk1 : Outport
  wires:
  Gain/1 -> Mux/1
  Temperature/1 -> R1/2, C1/2
  x/1 -> Get SOC/1, Get V1/1, Add/1
  Product/1 -> Add/2
  Add1/1 -> Mux/2  "xdot_2"
  Add/1 -> xk1/1
  Divide2/1 -> Add1/1
  Mux/1 -> Product/1  "xdot"
  Selector/1 -> Product/2
  Current/1 -> Probe/1, Divide1/1, Gain/1  "Current"
  C1/1 -> Divide1/2, Product1/2  "C1"
  Get V1/1 -> Divide2/1
  R1/1 -> Product1/1  "R1"
  Get SOC/1 -> R1/1, C1/1
  Product1/1 -> Divide2/2  "R1*C1"
  Divide1/1 -> Add1/2  "Current/C1"
  Probe/1 -> Selector/1

== system EV_Modeling_old/FV1/SOC Estimator (Kalman Filter)1/Kalman Filter/UKF 2RC/Prediction/Measurement function/Measurement function ==
  Current : Inport
  Temperature : Inport  Port=2
  x : Inport  Port=3
  Add2 : Sum  Inputs=+---
  Get SOC : Selector  InputPortWidth=3  IndexOptions=Index vector (dialog)  Indices=[1]  OutputSizes=1
  Get V1 : Selector  InputPortWidth=3  IndexOptions=Index vector (dialog)  Indices=2  OutputSizes=1
  Get V2 : Selector  InputPortWidth=3  IndexOptions=Index vector (dialog)  Indices=3  OutputSizes=1
  OCV Table : Lookup_n-D  BreakpointsForDimension1=SOC_vec  BreakpointsForDimension2=T_vec  BeginIndexSearchUsingPreviousIndexResult=on  Table=V0_mat  ExtrapMethod=Clip  InternalRulePriority=Speed  RndMeth=Simplest
      settings: InputPortMap=u0,u1
  Product2 : Product
  R0 Table : Lookup_n-D  BreakpointsForDimension1=SOC_vec  BreakpointsForDimension2=T_vec  BeginIndexSearchUsingPreviousIndexResult=on  Table=R0_mat  ExtrapMethod=Clip  InternalRulePriority=Speed  RndMeth=Simplest
      settings: InputPortMap=u0,u1
  y : Outport
  wires:
  Get V2/1 -> Add2/4  "V2"
  x/1 -> Get SOC/1, Get V1/1, Get V2/1
  OCV Table/1 -> Add2/1
  Current/1 -> Product2/2
  Get SOC/1 -> OCV Table/1, R0 Table/1
  Get V1/1 -> Add2/3  "V1"
  Product2/1 -> Add2/2
  Add2/1 -> y/1
  R0 Table/1 -> Product2/1
  Temperature/1 -> R0 Table/2, OCV Table/2

== system EV_Modeling_old/FV1/SOC Estimator (Kalman Filter)1/Kalman Filter/UKF 2RC/Prediction/State function/State function ==
  Current : Inport
  Temperature : Inport  Port=2
  x : Inport  Port=3
  Add : Sum
  Add1 : Sum  Inputs=-+
  Add2 : Sum  Inputs=-+
  C1 : Lookup_n-D  BreakpointsForDimension1=SOC_vec  BreakpointsForDimension2=T_vec  BeginIndexSearchUsingPreviousIndexResult=on  Table=C1_mat  ExtrapMethod=Clip  InternalRulePriority=Speed  RndMeth=Simplest
      settings: InputPortMap=u0,u1
  C2 : Lookup_n-D  BreakpointsForDimension1=SOC_vec  BreakpointsForDimension2=T_vec  Table=C2_mat  InternalRulePriority=Speed  RndMeth=Simplest
      settings: InputPortMap=u0,u1
  Divide{1..4} (4 alike) : Product  Inputs=*/
  Gain : Gain  Gain=-1/(AH*3600)
  Get SOC : Selector  InputPortWidth=3  IndexOptions=Index vector (dialog)  Indices=1  OutputSizes=1
  Get V1 : Selector  InputPortWidth=3  IndexOptions=Index vector (dialog)  Indices=2  OutputSizes=1
  Get V2 : Selector  InputPortWidth=3  IndexOptions=Index vector (dialog)  Indices=3  OutputSizes=1
  Mux : Mux  Inputs=3
  Probe : Probe  ProbeWidth=off  ProbeComplexSignal=off  ProbeSampleTimeDataType=Same as input
  Product : Product  OutDataTypeStr=single
  Product1 : Product
  Product2 : Product
  R1 : Lookup_n-D  BreakpointsForDimension1=SOC_vec  BreakpointsForDimension2=T_vec  BeginIndexSearchUsingPreviousIndexResult=on  Table=R1_mat  ExtrapMethod=Clip  InternalRulePriority=Speed  RndMeth=Simplest
      settings: InputPortMap=u0,u1
  R2 : Lookup_n-D  BreakpointsForDimension1=SOC_vec  BreakpointsForDimension2=T_vec  Table=R2_mat  InternalRulePriority=Speed  RndMeth=Simplest
      settings: InputPortMap=u0,u1
  Selector : Selector  InputPortWidth=2  IndexOptions=Index vector (dialog)  Indices=1  OutputSizes=1
  xk1 : Outport
  wires:
  Get V2/1 -> Divide3/1
  Add2/1 -> Mux/3  "xdot_3"
  Divide4/1 -> Add2/2  "Current/C2"
  Divide3/1 -> Add2/1
  Product2/1 -> Divide3/2  "R2*C2"
  C2/1 -> Product2/2, Divide4/2  "C2"
  R2/1 -> Product2/1  "R2"
  Gain/1 -> Mux/1
  Temperature/1 -> R1/2, C1/2, R2/2, C2/2
  x/1 -> Get SOC/1, Get V1/1, Add/1, Get V2/1
  Product/1 -> Add/2
  Add1/1 -> Mux/2  "xdot_2"
  Add/1 -> xk1/1
  Divide2/1 -> Add1/1
  Mux/1 -> Product/1  "xdot"
  Selector/1 -> Product/2
  Current/1 -> Probe/1, Divide1/1, Gain/1, Divide4/1  "Current"
  C1/1 -> Divide1/2, Product1/2  "C1"
  Get V1/1 -> Divide2/1
  R1/1 -> Product1/1  "R1"
  Get SOC/1 -> R1/1, C1/1, R2/1, C2/1
  Product1/1 -> Divide2/2  "R1*C1"
  Divide1/1 -> Add1/2  "Current/C1"
  Probe/1 -> Selector/1

== system EV_Modeling_old/FV2/SOC Estimator (Kalman Filter)1/Kalman Filter/UKBF/Prediction-correction/Measurement function/Measurement function ==
  Current : Inport
  Temperature : Inport  Port=2
  x : Inport  Port=3
  Add2 : Sum  Inputs=+--
  Get SOC1 : Selector  InputPortWidth=2  IndexOptions=Index vector (dialog)  Indices=[1]  OutputSizes=1
  Get V1 : Selector  InputPortWidth=2  IndexOptions=Index vector (dialog)  Indices=2  OutputSizes=1
  OCV Table : Lookup_n-D  BreakpointsForDimension1=SOC_vec  BreakpointsForDimension2=T_vec  BeginIndexSearchUsingPreviousIndexResult=on  Table=V0_mat  ExtrapMethod=Clip  InternalRulePriority=Speed  RndMeth=Simplest
      settings: InputPortMap=u0,u1
  Product2 : Product
  R0 Table : Lookup_n-D  BreakpointsForDimension1=SOC_vec  BreakpointsForDimension2=T_vec  BeginIndexSearchUsingPreviousIndexResult=on  Table=R0_mat  ExtrapMethod=Clip  InternalRulePriority=Speed  RndMeth=Simplest
      settings: InputPortMap=u0,u1
  y : Outport
  wires:
  x/1 -> Get SOC1/1, Get V1/1
  OCV Table/1 -> Add2/1
  Current/1 -> Product2/2
  Get SOC1/1 -> OCV Table/1, R0 Table/1  "SOC"
  Get V1/1 -> Add2/3
  Product2/1 -> Add2/2
  Add2/1 -> y/1
  R0 Table/1 -> Product2/1
  Temperature/1 -> R0 Table/2, OCV Table/2

== system EV_Modeling_old/FV2/SOC Estimator (Kalman Filter)1/Kalman Filter/UKBF/Prediction-correction/State function/State function ==
  Current : Inport
  Temperature : Inport  Port=2
  x : Inport  Port=3
  Add1 : Sum  Inputs=-+
  C1 : Lookup_n-D  BreakpointsForDimension1=SOC_vec  BreakpointsForDimension2=T_vec  BeginIndexSearchUsingPreviousIndexResult=on  Table=C1_mat  ExtrapMethod=Clip  InternalRulePriority=Speed  RndMeth=Simplest
      settings: InputPortMap=u0,u1
  Divide1 : Product  Inputs=*/
  Divide2 : Product  Inputs=*/
  Gain : Gain  Gain=-1/(AH*3600)
  Get SOC : Selector  InputPortWidth=2  IndexOptions=Index vector (dialog)  Indices=1  OutputSizes=1
  Get V1 : Selector  InputPortWidth=2  IndexOptions=Index vector (dialog)  Indices=2  OutputSizes=1
  Mux : Mux  Inputs=2
  Product1 : Product
  R1 : Lookup_n-D  BreakpointsForDimension1=SOC_vec  BreakpointsForDimension2=T_vec  BeginIndexSearchUsingPreviousIndexResult=on  Table=R1_mat  ExtrapMethod=Clip  InternalRulePriority=Speed  RndMeth=Simplest
      settings: InputPortMap=u0,u1
  f(x) : Outport
  wires:
  Gain/1 -> Mux/1
  Temperature/1 -> R1/2, C1/2
  x/1 -> Get SOC/1, Get V1/1
  Add1/1 -> Mux/2  "xdot_2"
  Divide2/1 -> Add1/1
  Mux/1 -> f(x)/1  "xdot"
  Current/1 -> Divide1/1, Gain/1  "Current"
  C1/1 -> Divide1/2, Product1/2  "C1"
  Get V1/1 -> Divide2/1  "V1"
  R1/1 -> Product1/1  "R1"
  Get SOC/1 -> R1/1, C1/1
  Product1/1 -> Divide2/2  "R1*C1"
  Divide1/1 -> Add1/2  "Current/C1"

== system EV_Modeling_old/FV2/SOC Estimator (Kalman Filter)1/Kalman Filter/UKBF/Prediction-correction/Xdot/Sigma points derivatives ==
  A : Inport
  Fi : Inport  Port=2
  x1 : Inport  Port=3
  Assignment : Assignment  NumberOfDimensions=2  DiagnosticForDimensions=Warning  IndexOptions=Index vector (dialog),Index vector (dialog)  Indices=1:n,1  OutputSizes=1,1
  Assignment1 : Assignment  NumberOfDimensions=2  DiagnosticForDimensions=Warning  IndexOptions=Index vector (dialog),Index vector (dialog)  Indices=1:n,2:n+1  OutputSizes=1,1
  Assignment2 : Assignment  NumberOfDimensions=2  DiagnosticForDimensions=Warning  IndexOptions=Index vector (dialog),Index vector (dialog)  Indices=1:n,n+2:2*n+1  OutputSizes=1,1
  Constant : Constant  Value=zeros(n,2*n+1)
  Constant1 : Constant  Value=ones(1,n)  VectorParams1D=off
  Gain : Gain  Gain=c_sqrt
  Matrix Multiply : Product  Multiplication=Matrix(*)
  Matrix Multiply1 : Product  Multiplication=Matrix(*)
  Sum : Sum  Inputs=|++
  Sum1 : Sum  Inputs=|+-
  Xdot : Outport
  wires:
  x1/1 -> Matrix Multiply/1, Assignment/2
  Constant1/1 -> Matrix Multiply/2
  Matrix Multiply/1 -> Sum1/1, Sum/1
  Gain/1 -> Sum1/2, Sum/2
  Sum/1 -> Assignment1/2
  Sum1/1 -> Assignment2/2
  Constant/1 -> Assignment/1
  Assignment/1 -> Assignment1/1
  Assignment1/1 -> Assignment2/1
  Assignment2/1 -> Xdot/1
  A/1 -> Matrix Multiply1/1
  Fi/1 -> Matrix Multiply1/2
  Matrix Multiply1/1 -> Gain/1

== system EV_Modeling_old/FV2/SOC Estimator (Kalman Filter)1/Kalman Filter/UKBF/Prediction-correction/Xdot/Update Fi ==
  A : Inport
  XWf : Inport  Port=2
  fWX : Inport  Port=3
  K : Inport  Port=4
  Constant1 : Constant  Value=double(Q)
  Constant4 : Constant  Value=eye(size(P0,1))
  Constant5 : Constant  Value=double(R)
  Divide1 : Product  Inputs=*/  Multiplication=Matrix(*)
  Gain5 : Gain  Gain=tril(ones(n)-diag(0.5*ones(1,n)))
  Matrix Multiply7 : Product  Inputs=3  Multiplication=Matrix(*)
  Matrix Multiply8 : Product  Inputs=3  Multiplication=Matrix(*)
  Sum3 : Sum  Inputs=+++-
  Transpose3 : Math  Operator=transpose
  Transpose4 : Math  Operator=transpose
  Fi : Outport
  wires:
  A/1 -> Divide1/2
  Matrix Multiply7/1 -> Gain5/1  "M"
  Constant1/1 -> Sum3/3
  Sum3/1 -> Matrix Multiply7/2
  Transpose3/1 -> Matrix Multiply8/3
  Matrix Multiply8/1 -> Sum3/4
  Divide1/1 -> Transpose4/1, Matrix Multiply7/1
  K/1 -> Transpose3/1, Matrix Multiply8/1
  XWf/1 -> Sum3/1
  Constant4/1 -> Divide1/1
  Transpose4/1 -> Matrix Multiply7/3
  Constant5/1 -> Matrix Multiply8/2
  fWX/1 -> Sum3/2
  Gain5/1 -> Fi/1  "Fi"

== system EV_Modeling_old/FV2/SOC Estimator (Kalman Filter)1/Kalman Filter/UKBF 2RC/Prediction-correction/Measurement function/Measurement function ==
  Current : Inport
  Temperature : Inport  Port=2
  x : Inport  Port=3
  Add2 : Sum  Inputs=+---
  Get SOC1 : Selector  InputPortWidth=3  IndexOptions=Index vector (dialog)  Indices=[1]  OutputSizes=1
  Get V1 : Selector  InputPortWidth=3  IndexOptions=Index vector (dialog)  Indices=2  OutputSizes=1
  Get V2 : Selector  InputPortWidth=3  IndexOptions=Index vector (dialog)  Indices=3  OutputSizes=1
  OCV Table : Lookup_n-D  BreakpointsForDimension1=SOC_vec  BreakpointsForDimension2=T_vec  BeginIndexSearchUsingPreviousIndexResult=on  Table=V0_mat  ExtrapMethod=Clip  InternalRulePriority=Speed  RndMeth=Simplest
      settings: InputPortMap=u0,u1
  Product2 : Product
  R0 Table : Lookup_n-D  BreakpointsForDimension1=SOC_vec  BreakpointsForDimension2=T_vec  BeginIndexSearchUsingPreviousIndexResult=on  Table=R0_mat  ExtrapMethod=Clip  InternalRulePriority=Speed  RndMeth=Simplest
      settings: InputPortMap=u0,u1
  y : Outport
  wires:
  Get V2/1 -> Add2/4
  x/1 -> Get SOC1/1, Get V1/1, Get V2/1
  OCV Table/1 -> Add2/1
  Current/1 -> Product2/2
  Get SOC1/1 -> OCV Table/1, R0 Table/1  "SOC"
  Get V1/1 -> Add2/3
  Product2/1 -> Add2/2
  Add2/1 -> y/1
  R0 Table/1 -> Product2/1
  Temperature/1 -> R0 Table/2, OCV Table/2

== system EV_Modeling_old/FV2/SOC Estimator (Kalman Filter)1/Kalman Filter/UKBF 2RC/Prediction-correction/State function/State function ==
  Current : Inport
  Temperature : Inport  Port=2
  x : Inport  Port=3
  2-D Lookup Table C2 : Lookup_n-D  BreakpointsForDimension1=SOC_vec  BreakpointsForDimension2=T_vec  Table=C2_mat  InternalRulePriority=Speed  RndMeth=Simplest
      settings: InputPortMap=u0,u1
  2-D Lookup Table R2 : Lookup_n-D  BreakpointsForDimension1=SOC_vec  BreakpointsForDimension2=T_vec  Table=R2_mat  InternalRulePriority=Speed  RndMeth=Simplest
      settings: InputPortMap=u0,u1
  Add1 : Sum  Inputs=-+
  Add2 : Sum  Inputs=-+
  C1 : Lookup_n-D  BreakpointsForDimension1=SOC_vec  BreakpointsForDimension2=T_vec  BeginIndexSearchUsingPreviousIndexResult=on  Table=C1_mat  ExtrapMethod=Clip  InternalRulePriority=Speed  RndMeth=Simplest
      settings: InputPortMap=u0,u1
  Divide{1..4} (4 alike) : Product  Inputs=*/
  Gain : Gain  Gain=-1/(AH*3600)
  Get SOC : Selector  InputPortWidth=3  IndexOptions=Index vector (dialog)  Indices=1  OutputSizes=1
  Get V1 : Selector  InputPortWidth=3  IndexOptions=Index vector (dialog)  Indices=2  OutputSizes=1
  Get V2 : Selector  InputPortWidth=3  IndexOptions=Index vector (dialog)  Indices=3  OutputSizes=1
  Mux : Mux  Inputs=3
  Product1 : Product
  Product2 : Product
  R1 : Lookup_n-D  BreakpointsForDimension1=SOC_vec  BreakpointsForDimension2=T_vec  BeginIndexSearchUsingPreviousIndexResult=on  Table=R1_mat  ExtrapMethod=Clip  InternalRulePriority=Speed  RndMeth=Simplest
      settings: InputPortMap=u0,u1
  f(x) : Outport
  wires:
  Divide4/1 -> Add2/2  "Current/C2"
  Divide3/1 -> Add2/1
  Add2/1 -> Mux/3  "xdot_3"
  Product2/1 -> Divide3/2  "R1*C1"
  Get V2/1 -> Divide3/1  "V2"
  2-D Lookup Table C2/1 -> Product2/2, Divide4/2  "C2"
  2-D Lookup Table R2/1 -> Product2/1  "R2"
  Gain/1 -> Mux/1
  Temperature/1 -> R1/2, C1/2, 2-D Lookup Table R2/2, 2-D Lookup Table C2/2
  x/1 -> Get SOC/1, Get V1/1, Get V2/1
  Add1/1 -> Mux/2  "xdot_2"
  Divide2/1 -> Add1/1
  Mux/1 -> f(x)/1  "xdot"
  Current/1 -> Divide1/1, Gain/1, Divide4/1  "Current"
  C1/1 -> Divide1/2, Product1/2  "C1"
  Get V1/1 -> Divide2/1  "V1"
  R1/1 -> Product1/1  "R1"
  Get SOC/1 -> R1/1, C1/1, 2-D Lookup Table R2/1, 2-D Lookup Table C2/1
  Product1/1 -> Divide2/2  "R1*C1"
  Divide1/1 -> Add1/2  "Current/C1"
